simulink model "prac1cain"  (R2023a)
settings: Solver=VariableStepAuto  StartTime=0.0  StopTime=10.0  RelTol=1e-3
settings Model: Creator=User  LastModifiedBy=User

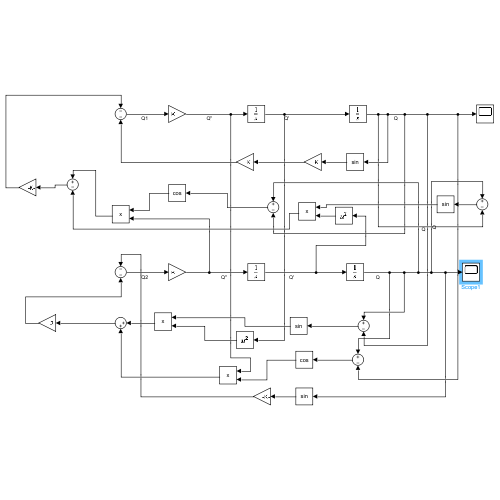
[thumbnail: Simulink's stored preview of the top-level diagram]
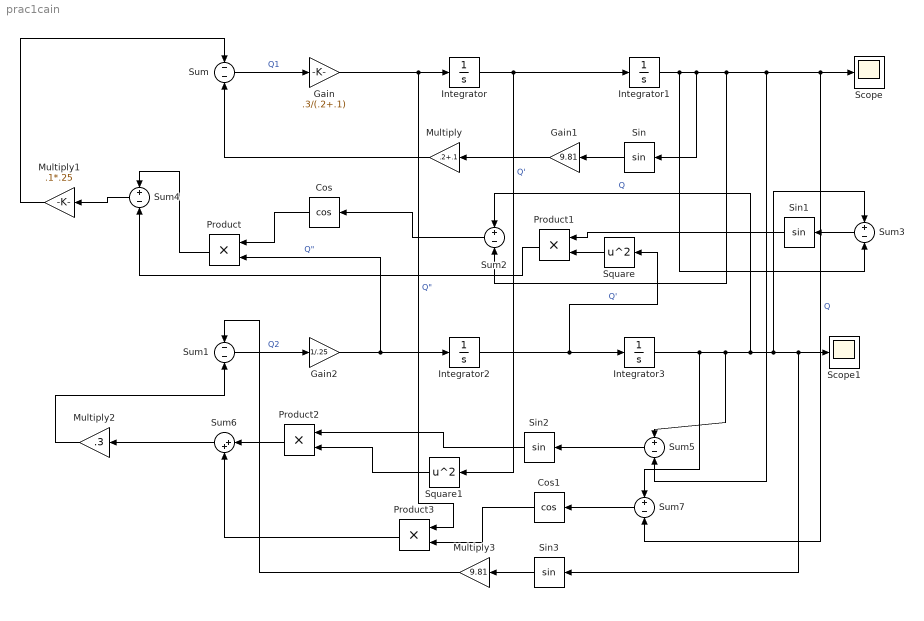
== system prac1cain ==
  Cos : Trigonometry  Operator=cos
  Cos1 : Trigonometry  Operator=cos
  Gain : Gain  Gain=.3/(.2+.1)
  Gain1 : Gain  Gain=9.81
  Gain2 : Gain  Gain=1/.25
  Integrator : Integrator
  Integrator1 : Integrator
  Integrator2 : Integrator
  Integrator3 : Integrator  InitialCondition=35*(pi/180)
  Multiply : Gain  Gain=.2+.1
  Multiply1 : Gain  Gain=.1*.25
  Multiply2 : Gain  Gain=.3
  Multiply3 : Gain  Gain=9.81
  Product{,1..3} (4 alike) : Product
  Scope : Scope
  Scope1 : Scope
  Sin{,1..3} (4 alike) : Trigonometry
  Square : Math  Operator=square
  Square1 : Math  Operator=square
  Sum : Sum  Inputs=--
  Sum1 : Sum  Inputs=--
  Sum{2..5,7} (5 alike) : Sum  Inputs=+-
  Sum6 : Sum  Inputs=|++
  wires:
  Integrator/1 -> Integrator1/1, Square1/1  "Q'"
  Sum/1 -> Gain/1  "Q1"
  Gain/1 -> Product3/1, Integrator/1  "Q\""
  Sin/1 -> Gain1/1
  Integrator1/1 -> Sum3/2, Sum5/2, Sum7/2, Scope/1, Sum2/2, Sin/1  "Q"
  Sum1/1 -> Gain2/1  "Q2"
  Gain2/1 -> Product/2, Integrator2/1  "Q\""
  Integrator2/1 -> Square/1, Integrator3/1  "Q'"
  Integrator3/1 -> Sum7/1, Sum5/1, Sin3/1, Scope1/1, Sum3/1, Sum2/1  "Q"
  Sum2/1 -> Cos/1
  Cos/1 -> Product/1
  Gain1/1 -> Multiply/1
  Sum3/1 -> Sin1/1
  Square/1 -> Product1/2
  Sin1/1 -> Product1/1
  Product/1 -> Sum4/1
  Product1/1 -> Sum4/2
  Sum4/1 -> Multiply1/1
  Multiply1/1 -> Sum/1
  Multiply/1 -> Sum/2
  Sum5/1 -> Sin2/1
  Square1/1 -> Product2/2
  Sin2/1 -> Product2/1
  Product2/1 -> Sum6/1
  Sum7/1 -> Cos1/1
  Cos1/1 -> Product3/2
  Product3/1 -> Sum6/2
  Sum6/1 -> Multiply2/1
  Multiply2/1 -> Sum1/2
  Sin3/1 -> Multiply3/1
  Multiply3/1 -> Sum1/1
